simulink model "DC_Motor_HIL"  (R2018b)
settings: Solver=FixedStepAuto  StartTime=0.0  StopTime=inf  FixedStep=0.004  RelTol=1e-3
undefined symbols (not defined in the file or in its folder): Hc_DC
settings Model: SimulationMode=external  ExtModeTrigDuration=200  Creator=young  LastModifiedBy=root
settings DataIOCC: SaveOutput=off  SaveTime=off
settings OptimizationCC: EnhancedBackFolding=on  PassReuseOutputArgsAs=Individual arguments  OptimizeBlockOrder=speed  DifferentSizesBufferReuse=on  OptimizationCustomize=off
settings DebuggingCC: ParameterTunabilityLossMsg=error
settings HardwareCC: ProdBitPerPointer=32  ProdBitPerSizeT=32  ProdBitPerPtrDiffT=32  ProdLargestAtomicInteger=Integer  ProdLargestAtomicFloat=None  ProdWordSize=32  ProdLongLongMode=on  ProdHWDeviceType=Custom Processor
settings SFSimCC: SimUseLocalCustomCode=off  MATLABDynamicMemAlloc=off
settings RTWCC: SystemTargetFile=CompSOC_ec.tlc  TemplateMakefile=CompSOC_ec.tmf  Description=CompSOC EC Target  RTWUseLocalCustomCode=off  IncludeHyperlinkInReport=on  CodeExecutionProfiling=on  CodeProfilingSaveOptions=AllData  CodeProfilingInstrumentation=detailed
settings CodeAppCC: ForceParamTrailComments=on  IgnoreCustomStorageClasses=off  OperatorAnnotations=on  SimulinkDataObjDesc=on  SFDataObjDesc=on  InsertBlockDesc=on
settings STFCustomTargetCC: TargetLibSuffix=.a  TargetLangStandard=C99 (ISO)  MultiwordLength=256  GenerateSampleERTMain=on  CombineOutputUpdateFcns=on  ERTCustomFileBanners=on  SupportNonInlinedSFcns=off  RemoveResetFunc=on  MATLABClassNameForMDSCustomization=Simulink.SoftwareTarget.ERTCustomization  SystemTargetFile=CompSOC_ec.tlc
settings ERTTargetCC: TargetLangStandard=C99 (ISO)  GenerateSampleERTMain=on  ParMdlRefBuildCompliant=off  CompOptLevelCompliant=off  ConcurrentExecutionCompliant=off  SupportContinuousTime=on  ModelStepFunctionPrototypeControlCompliant=off  CPPClassGenCompliant=off  UseToolchainInfoCompliant=off  ExtMode=on  ExtModeStaticAlloc=on  ExtModeStaticAllocSize=9200  ExtModeMexArgs='pato-board.local' 1 9879  ERTCustomFileTemplate=CompSOC_ec_file_process.tlc

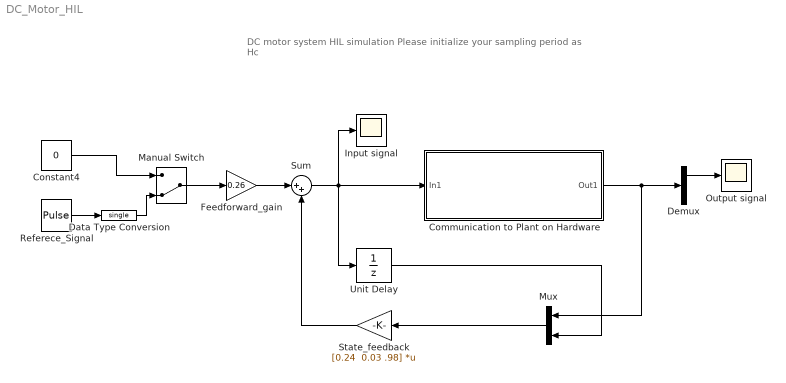
== system DC_Motor_HIL ==
  note: DC motor system HIL simulation
      | Please initialize your sampling period as Hc
  Communication to Plant on Hardware : Subsystem
  Constant4 : Constant  Value=0  OutDataTypeStr=single  SampleTime=Hc_DC
  Data Type Conversion : DataTypeConversion  OutDataTypeStr=single
  Demux : Demux  Outputs=2
  Feedforward_gain : Gain  Gain=0.26
  Input signal : Scope
  Manual Switch : ManualSwitch  CurrentSetting=0
  Mux : Mux  Inputs=2
  Output signal : Scope
  Referece_Signal : DiscretePulseGenerator  Period=2500  PulseWidth=1250  SampleTime=Hc_DC
  State_feedback : Gain  Gain="[0.24  0.03 .98]"  Multiplication=Matrix(K*u) (u vector)
  Sum : Sum  Inputs=|++
  Unit Delay : UnitDelay  SampleTime=Hc_DC
  wires:
  Sum/1 -> Unit Delay/1, Communication to Plant on Hardware/1(In1), Input signal/1
  Feedforward_gain/1 -> Sum/1
  State_feedback/1 -> Sum/2
  Manual Switch/1 -> Feedforward_gain/1
  Constant4/1 -> Manual Switch/1
  Unit Delay/1 -> Mux/2
  Data Type Conversion/1 -> Manual Switch/2
  Referece_Signal/1 -> Data Type Conversion/1
  Mux/1 -> State_feedback/1
  Demux/1 -> Output signal/1
  Communication to Plant on Hardware/1(Out1) -> Mux/1, Demux/1

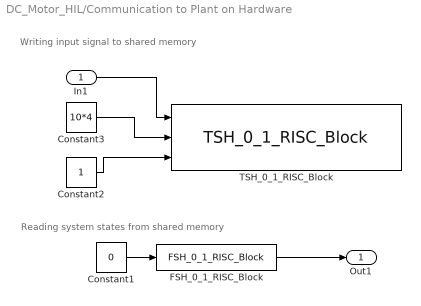
== system DC_Motor_HIL/Communication to Plant on Hardware ==
  note: Reading system states from shared memory
  note: Writing input signal to shared memory
  In1 : Inport
  Constant1 : Constant  Value=0  OutDataTypeStr=int32  SampleTime=Hc_DC
  Constant2 : Constant  OutDataTypeStr=int32  SampleTime=Hc_DC
  Constant3 : Constant  Value=10*4  OutDataTypeStr=uint32  SampleTime=Hc_DC
  FSH_0_1_RISC_Block : S-Function  FunctionName=FSH_0_1_RISC_Block  Parameters=SParameter1  SFunctionDeploymentMode=off  EnableBusSupport=off  mask(Legacy Function){SFunctionSpec=void read(single y1[p1],int32 u1,int32 p1), SParameter1=2, ShowSpec=off}
      mask prompts: SParameter1 "P1:"; ShowSpec "Display function specification"
      mask help:
      | This block allows you to call the legacy functions specified by the following Legacy Code Tool definition:
      | def.SFunctionName = 'FSH_0_1_RISC_Block';
      | def.OutputFcnSpec = 'void read(single y1[p1],int32 u1,int32 p1)';
      | def.HeaderFiles = {'FSH_0_1_RISC.h'};
      mask Help: <p>This block was generated automatically by the Legacy Code Tool. For detailed help on this tool, call<a href="matlab:legacy_code('help')"> legacy_code('help')</a>.</p>
      mask Callback ShowSpec:
      | if strcmp(get_param(gcbh, 'ShowSpec'), 'on')
      |   set_param(gcbh, 'MaskDisplay', sprintf('fprintf(''%s'');', get_param(gcbh, 'SFunctionSpec')));
      | else
      |   set_param(gcbh, 'MaskDisplay', sprintf('fprintf(''%s'');', get_param(gcbh, 'FunctionName')));
      | end
      mask Display: fprintf('FSH_0_1_RISC_Block');
  TSH_0_1_RISC_Block : S-Function  FunctionName=TSH_0_1_RISC_Block  SFunctionDeploymentMode=off  EnableBusSupport=off  mask(Legacy Function){SFunctionSpec=write(single u1[], uint32 u2, int32 u3), ShowSpec=off}
      mask prompts: ShowSpec "Display function specification"
      mask help:
      | This block allows you to call the legacy functions specified by the following Legacy Code Tool definition:
      | def.SFunctionName = 'TSH_0_1_RISC_Block';
      | def.OutputFcnSpec = 'write(single u1[], uint32 u2, int32 u3)';
      | def.HeaderFiles = {'TSH_0_1_RISC.h'};
      mask Help: <p>This block was generated automatically by the Legacy Code Tool. For detailed help on this tool, call<a href="matlab:legacy_code('help')"> legacy_code('help')</a>.</p>
      mask Callback ShowSpec:
      | if strcmp(get_param(gcbh, 'ShowSpec'), 'on')
      |   set_param(gcbh, 'MaskDisplay', sprintf('fprintf(''%s'');', get_param(gcbh, 'SFunctionSpec')));
      | else
      |   set_param(gcbh, 'MaskDisplay', sprintf('fprintf(''%s'');', get_param(gcbh, 'FunctionName')));
      | end
      mask Display: fprintf('TSH_0_1_RISC_Block');
  Out1 : Outport
  wires:
  Constant2/1 -> TSH_0_1_RISC_Block/3
  FSH_0_1_RISC_Block/1 -> Out1/1
  In1/1 -> TSH_0_1_RISC_Block/1
  Constant1/1 -> FSH_0_1_RISC_Block/1
  Constant3/1 -> TSH_0_1_RISC_Block/2
